simulink model "CIC_Filter_R128_N5"  (R2022b)
settings: Solver=FixedStepAuto  StartTime=0.0  StopTime=10.0  FixedStep=Ts  RelTol=1e-3
model workspace (MAT data in the model file):
  Ts = 5e-07
settings Model: Creator=Rio  LastModifiedBy=Rio

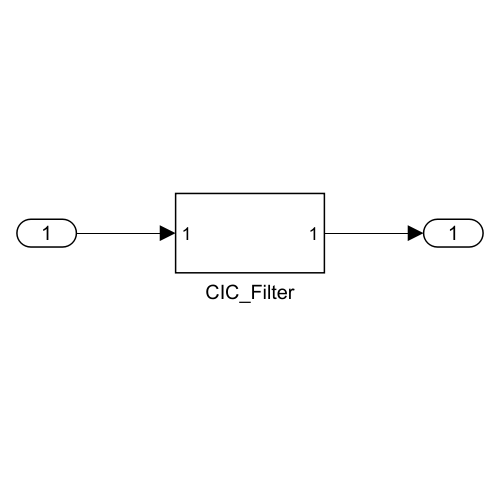
[thumbnail: Simulink's stored preview of the top-level diagram]
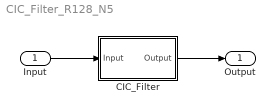
== system CIC_Filter_R128_N5 ==
  Input : Inport
  CIC_Filter : Subsystem  Tag=FilterWizardSubSystem
      settings: ErrorFcn=dspFilterRealizedInBasicElemsAlgLoopErrFcnCallback
  Output : Outport
  wires:
  Input/1 -> CIC_Filter/1(Input)
  CIC_Filter/1(Output) -> Output/1

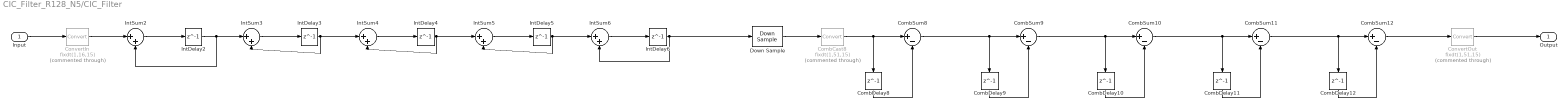
== system CIC_Filter_R128_N5/CIC_Filter ==
  Input : Inport
  CombCast8 : DataTypeConversion  Commented=through  OutDataTypeStr=fixdt(1,51,15)  SaturateOnIntegerOverflow=off  RndMeth=Floor
  CombDelay{8..12} (5 alike) : Delay  DelayLength=1  InitialCondition=0
  CombSum{8..12} (5 alike) : Sum  Inputs=|+-  AccumDataTypeStr=fixdt(1,51,15)  OutDataTypeStr=fixdt(1,51,15)
  ConvertIn : DataTypeConversion  Commented=through  OutDataTypeStr=fixdt(1,16,15)  RndMeth=Nearest
  ConvertOut : DataTypeConversion  Commented=through  OutDataTypeStr=fixdt(1,51,15)  SaturateOnIntegerOverflow=off  RndMeth=Floor
  Down Sample : DownSample  N=128  RateOptions=Allow multirate processing  AllowArbitraryFixedInput=on
  IntDelay{2..3,5..6} (4 alike) : Delay  DelayLength=1  InitialCondition=0  SampleTime=Ts
  IntDelay4 : Delay  DelayLength=1  InitialCondition=0
  IntSum{2..6} (5 alike) : Sum  Inputs=|++  AccumDataTypeStr=fixdt(1,51,15)  OutDataTypeStr=fixdt(1,51,15)
  Output : Outport
  wires:
  Input/1 -> ConvertIn/1
  ConvertIn/1 -> IntSum2/1
  IntSum2/1 -> IntDelay2/1
  IntDelay2/1 -> IntSum2/2, IntSum3/1
  IntSum3/1 -> IntDelay3/1
  IntDelay3/1 -> IntSum3/2, IntSum4/1
  IntSum4/1 -> IntDelay4/1
  IntDelay4/1 -> IntSum4/2, IntSum5/1
  IntSum5/1 -> IntDelay5/1
  IntDelay5/1 -> IntSum5/2, IntSum6/1
  IntSum6/1 -> IntDelay6/1
  IntDelay6/1 -> IntSum6/2, Down Sample/1
  Down Sample/1 -> CombCast8/1
  CombSum8/1 -> CombSum9/1, CombDelay9/1
  CombDelay8/1 -> CombSum8/2
  CombCast8/1 -> CombSum8/1, CombDelay8/1
  CombSum9/1 -> CombSum10/1, CombDelay10/1
  CombDelay9/1 -> CombSum9/2
  CombSum10/1 -> CombSum11/1, CombDelay11/1
  CombDelay10/1 -> CombSum10/2
  CombSum11/1 -> CombSum12/1, CombDelay12/1
  CombDelay11/1 -> CombSum11/2
  CombDelay12/1 -> CombSum12/2
  CombSum12/1 -> ConvertOut/1
  ConvertOut/1 -> Output/1
